simulink model "Simulation_VR"  (R2023a)
settings: Solver=VariableStepAuto  StartTime=0.0  StopTime=15  RelTol=1e-6
values from neighbouring files (symbols this model uses):
  a1 = 1    [main_RR_VR.m]
  a2 = 1    [main_RR_VR.m]
  b = 0.1    [main_RR_VR.m]
  dq0 = [0.0 ; 0.0]    [main_RR_VR.m]
  dq0_d = [0.0; 0.0]    [main_RR_VR.m]
  Il = (1/3)*m1*a1^2    (= 1.66666666667)    [main_RR_VR.m]
  Im = 740e-6    (= 0.00074)    [main_RR_VR.m]
  k_mot = 0.23    [main_RR_VR.m]
  K_pid = 5    [main_RR_VR.m]
  L = 50e-6    (= 5e-05)    [main_RR_VR.m]
  params = [a1, a2, m1, m2, l1, l2, Izz1, Izz2]    [main_RR_VR.m]
  q0 = [0.25 ; 0.25]    [main_RR_VR.m]
  q0_d = [pi/2; -pi/2]    [main_RR_VR.m]
  R = 0.11    [main_RR_VR.m]
  U = diag([1;1; u_min + rand([6,1])*(u_max - u_min)])    [main_RR_VR.m]
undefined symbols (not defined in the file or in its folder): Ks, Lambda, rel_err
settings Model: Creator=Mathew  LastModifiedBy=rvitt
settings SolverCC: AlgebraicLoopSolver=TrustRegion
settings OptimizationCC: ReuseModelBlockBuffer=off
settings DebuggingCC: UnconnectedInputMsg=warning  UnconnectedOutputMsg=warning  UnconnectedLineMsg=warning  ArithmeticOperatorsInVariantConditions=warning
settings ModelReferenceCC: EnableRefExpFcnMdlSchedulingChecks=on
settings SFSimCC: CustomCodeUndefinedFunction=UseInterfaceOnly

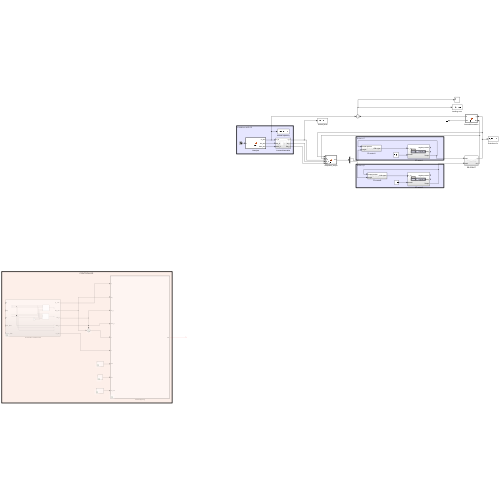
[thumbnail: Simulink's stored preview of the top-level diagram]
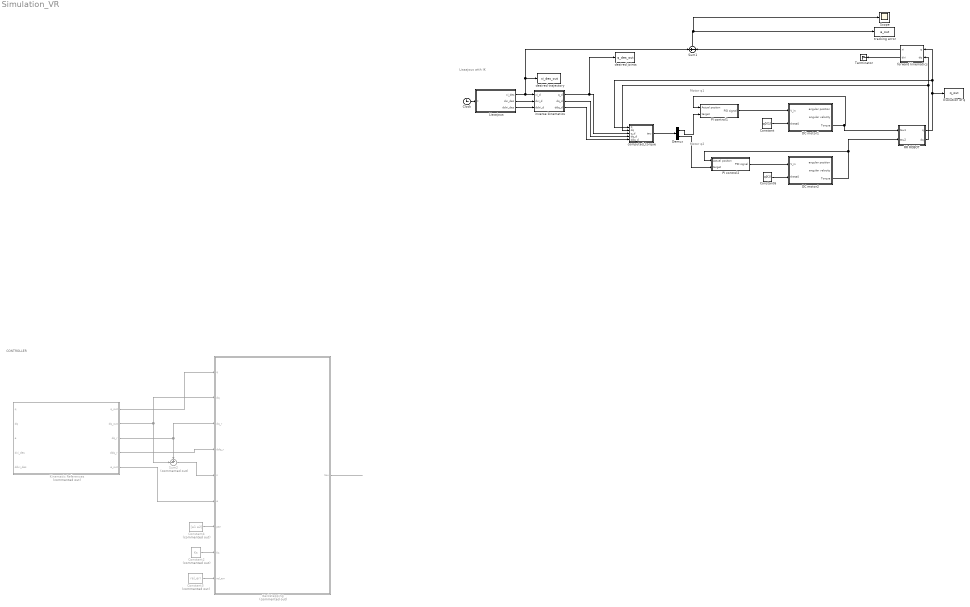
== system Simulation_VR ==
  note: Lissajous with IK
  note: CONTROLLER
  note: Motor q1
  note: Motor q2
  Backstepping : MATLAB Function  Commented=on  TreatAsAtomicUnit=on
  Clock : Clock
  Constant : Constant  Value=q0(1)
  Constant2 : Constant  Commented=on  Value=Ks
  Constant3 : Constant  Commented=on  Value=rel_err
  Constant4 : Constant  Commented=on  Value=[a1 a2]
  Constant6 : Constant  Value=q0(2)
  DC motor1 : Subsystem
  DC motor2 : Subsystem
  Demux : Demux  Outputs=2
  Evolution of q : ToWorkspace  VariableName=q_out  SaveFormat=Timeseries  SampleTime=-1
  Kinematic References : Subsystem  Commented=on
  Lissajous : MATLAB Function  TreatAsAtomicUnit=on
  PI control1 : Subsystem
  PI control2 : Subsystem
  RR ROBOT : Subsystem
  Scope : Scope
  Sum1 : Sum  Inputs=+-
  Sum2 : Sum  Commented=on  Inputs=+-|
  Terminator : Terminator
  computed_torque : MATLAB Function  TreatAsAtomicUnit=on
  desired joints : ToWorkspace  VariableName=q_des_out  SaveFormat=Timeseries  SampleTime=-1
  desired trajectory : ToWorkspace  VariableName=xi_des_out  SaveFormat=Timeseries  SampleTime=-1
  forward kinematics : MATLAB Function  TreatAsAtomicUnit=on
  inverse kinematics : Subsystem
  tracking error : ToWorkspace  VariableName=e_out  SaveFormat=Timeseries  SampleTime=-1
  wires:
  RR ROBOT/1(q) -> computed_torque/1(q), forward kinematics/1(q), Evolution of q/1
  Kinematic References/5(e_out) -> Backstepping/6(e)
  Kinematic References/3(dq_r) -> Backstepping/3(dq_r), Sum2/1
  Constant3/1 -> Backstepping/9(rel_err)
  Kinematic References/2(dq_out) -> Sum2/2, Backstepping/2(dq)
  Kinematic References/1("q_out ") -> Backstepping/1(q)
  Kinematic References/4(ddq_r) -> Backstepping/4(ddq_r)
  Sum2/1 -> Backstepping/5(s)
  Backstepping/1(tau) -> ?
  Constant2/1 -> Backstepping/8(Ks)
  Constant4/1 -> Backstepping/7(par)
  RR ROBOT/2(dq) -> computed_torque/2(dq), forward kinematics/2(dq)
  inverse kinematics/1(q_d) -> computed_torque/3(q_d), desired joints/1
  Clock/1 -> Lissajous/1(t)
  Lissajous/2(dxi_des) -> inverse kinematics/2(dxi_d)
  Lissajous/3(ddxi_des) -> inverse kinematics/3(ddxi_d)
  Lissajous/1(xi_des) -> Sum1/1, desired trajectory/1, inverse kinematics/1(xi_d)
  Sum1/1 -> Scope/1, tracking error/1
  forward kinematics/2(dxi) -> Terminator/1
  forward kinematics/1(xi) -> Sum1/2
  computed_torque/1(tau) -> Demux/1
  inverse kinematics/2(dq_d) -> computed_torque/4(dq_d)
  inverse kinematics/3(ddq_d) -> computed_torque/5(ddq_d)
  PI control1/1(PID signal) -> DC motor1/1(V_in)
  PI control2/1(PID signal) -> DC motor2/1(V_in)
  DC motor1/3(Torque) -> RR ROBOT/1(tau1), PI control1/1(Actual positon)
  Constant/1 -> DC motor1/2(theta0)
  Constant6/1 -> DC motor2/2(theta0)
  DC motor2/3(Torque) -> RR ROBOT/2(tau2), PI control2/1(Actual positon)
  Demux/2 -> PI control2/2(target)
  Demux/1 -> PI control1/2(target)

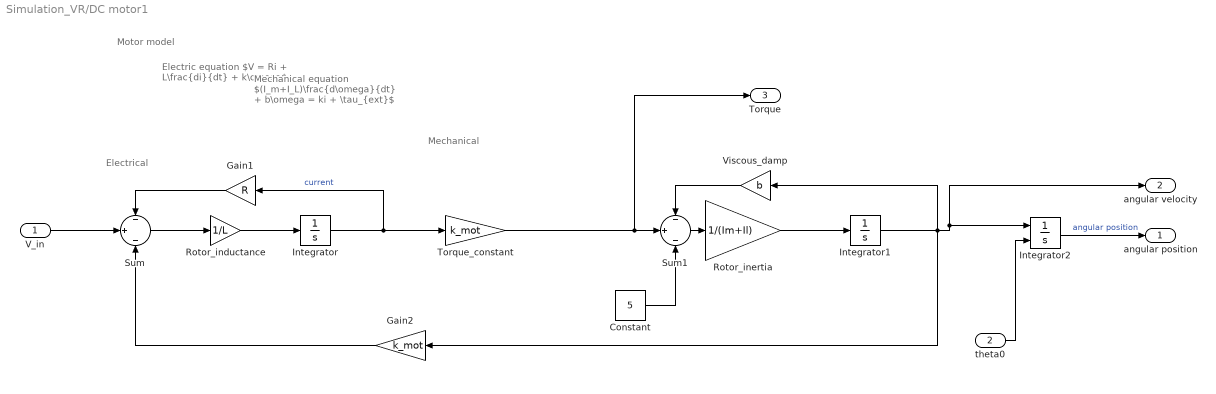
== system Simulation_VR/DC motor1 ==
  note: Electric equation
      | $V = Ri + L\frac{di}{dt} + k\omega$
  note: Mechanical equation
      | $(I_m+I_L)\frac{d\omega}{dt} + b\omega = ki + \tau_{ext}$
  note: Motor model
  note: Electrical
  note: Mechanical
  V_in : Inport
  theta0 : Inport  Port=2
  Constant : Constant  Value=5
  Gain1 : Gain  Gain=R
  Gain2 : Gain  Gain=k_mot
  Integrator : Integrator
  Integrator1 : Integrator
  Integrator2 : Integrator  InitialConditionSource=external
  Rotor_inductance : Gain  Gain=1/L
  Rotor_inertia : Gain  Gain=1/(Im+Il)
  Sum : Sum  Inputs=-|+|-
  Sum1 : Sum  Inputs=-|+|-
  Torque_constant : Gain  Gain=k_mot
  Viscous_damp : Gain  Gain=b
  angular position : Outport
  angular velocity : Outport  Port=2
  Torque : Outport  Port=3
  wires:
  theta0/1 -> Integrator2/2
  Integrator1/1 -> Gain2/1, Integrator2/1, angular velocity/1, Viscous_damp/1
  Torque_constant/1 -> Sum1/2, Torque/1
  Integrator2/1 -> angular position/1  "angular position"
  Gain2/1 -> Sum/3
  Gain1/1 -> Sum/1
  Rotor_inertia/1 -> Integrator1/1
  V_in/1 -> Sum/2
  Rotor_inductance/1 -> Integrator/1
  Sum1/1 -> Rotor_inertia/1
  Viscous_damp/1 -> Sum1/1
  Integrator/1 -> Torque_constant/1, Gain1/1  "current"
  Sum/1 -> Rotor_inductance/1
  Constant/1 -> Sum1/3

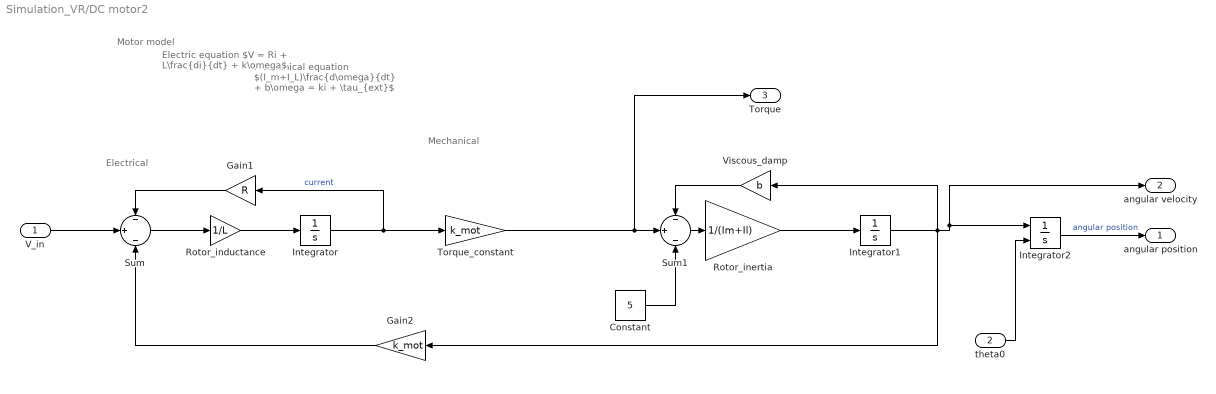
== system Simulation_VR/DC motor2 ==
  note: Mechanical
  note: Electrical
  note: Motor model
  note: Mechanical equation
      | $(I_m+I_L)\frac{d\omega}{dt} + b\omega = ki + \tau_{ext}$
  note: Electric equation
      | $V = Ri + L\frac{di}{dt} + k\omega$
  V_in : Inport
  theta0 : Inport  Port=2
  Constant : Constant  Value=5
  Gain1 : Gain  Gain=R
  Gain2 : Gain  Gain=k_mot
  Integrator : Integrator
  Integrator1 : Integrator
  Integrator2 : Integrator  InitialConditionSource=external
  Rotor_inductance : Gain  Gain=1/L
  Rotor_inertia : Gain  Gain=1/(Im+Il)
  Sum : Sum  Inputs=-|+|-
  Sum1 : Sum  Inputs=-|+|-
  Torque_constant : Gain  Gain=k_mot
  Viscous_damp : Gain  Gain=b
  angular position : Outport
  angular velocity : Outport  Port=2
  Torque : Outport  Port=3
  wires:
  Sum/1 -> Rotor_inductance/1
  Integrator/1 -> Gain1/1, Torque_constant/1  "current"
  Viscous_damp/1 -> Sum1/1
  Sum1/1 -> Rotor_inertia/1
  Rotor_inductance/1 -> Integrator/1
  V_in/1 -> Sum/2
  Rotor_inertia/1 -> Integrator1/1
  Gain1/1 -> Sum/1
  Gain2/1 -> Sum/3
  Integrator2/1 -> angular position/1  "angular position"
  Torque_constant/1 -> Torque/1, Sum1/2
  Integrator1/1 -> Viscous_damp/1, angular velocity/1, Integrator2/1, Gain2/1
  theta0/1 -> Integrator2/2
  Constant/1 -> Sum1/3

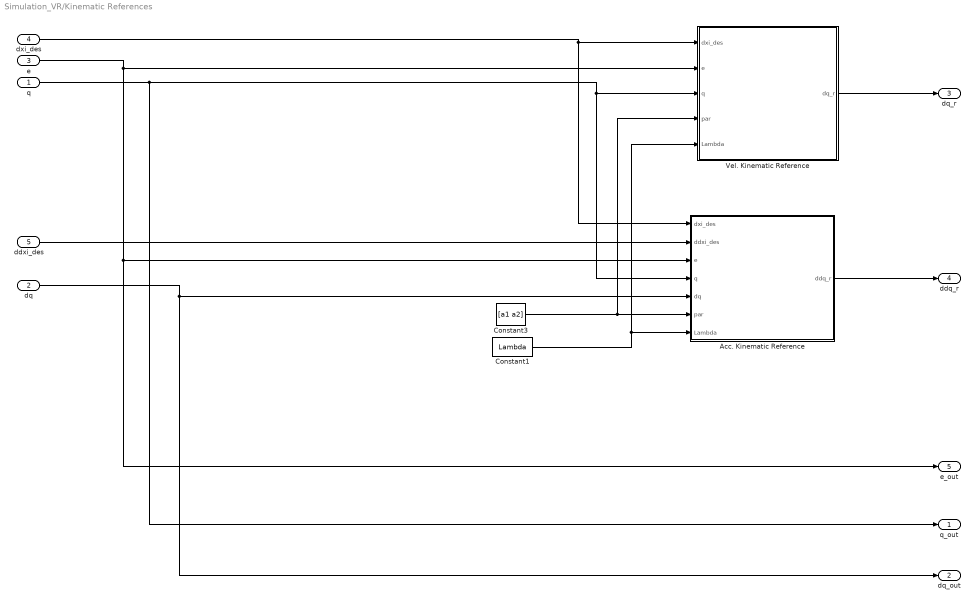
== system Simulation_VR/Kinematic References ==
  q : Inport
  dq : Inport  Port=2
  e : Inport  Port=3
  dxi_des : Inport  Port=4
  ddxi_des : Inport  Port=5
  Acc. Kinematic Reference : MATLAB Function  TreatAsAtomicUnit=on
  Constant1 : Constant  Value=Lambda
  Constant3 : Constant  Value=[a1 a2]
  "Vel. Kinematic Reference " : MATLAB Function  TreatAsAtomicUnit=on
  "q_out " : Outport  VectorParamsAs1DForOutWhenUnconnected=off
  dq_out : Outport  Port=2  VectorParamsAs1DForOutWhenUnconnected=off
  dq_r : Outport  Port=3  VectorParamsAs1DForOutWhenUnconnected=off
  ddq_r : Outport  Port=4  VectorParamsAs1DForOutWhenUnconnected=off
  e_out : Outport  Port=5  VectorParamsAs1DForOutWhenUnconnected=off
  wires:
  ddxi_des/1 -> Acc. Kinematic Reference/2(ddxi_des)
  e/1 -> e_out/1, Acc. Kinematic Reference/3(e), "Vel. Kinematic Reference "/2(e)
  dxi_des/1 -> Acc. Kinematic Reference/1(dxi_des), "Vel. Kinematic Reference "/1(dxi_des)
  Constant1/1 -> "Vel. Kinematic Reference "/5(Lambda), Acc. Kinematic Reference/7(Lambda)
  "Vel. Kinematic Reference "/1(dq_r) -> dq_r/1
  dq/1 -> dq_out/1, Acc. Kinematic Reference/5(dq)
  q/1 -> "q_out "/1, Acc. Kinematic Reference/4(q), "Vel. Kinematic Reference "/3(q)
  Constant3/1 -> "Vel. Kinematic Reference "/4(par), Acc. Kinematic Reference/6(par)
  Acc. Kinematic Reference/1(ddq_r) -> ddq_r/1

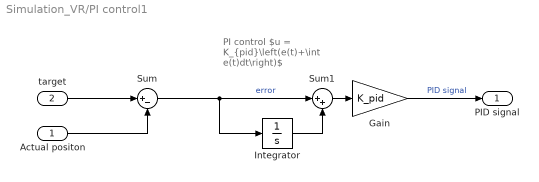
== system Simulation_VR/PI control1 ==
  note: PI control
      | $u = K_{pid}\left(e(t)+\int e(t)dt\right)$
  Actual positon : Inport
  target : Inport  Port=2
  Gain : Gain  Gain=K_pid
  Integrator : Integrator
  Sum : Sum  Inputs=|+-
  Sum1 : Sum  Inputs=|++
  PID signal : Outport
  wires:
  Actual positon/1 -> Sum/2
  Sum1/1 -> Gain/1
  Gain/1 -> PID signal/1  "PID signal"
  Sum/1 -> Integrator/1, Sum1/1  "error"
  target/1 -> Sum/1
  Integrator/1 -> Sum1/2

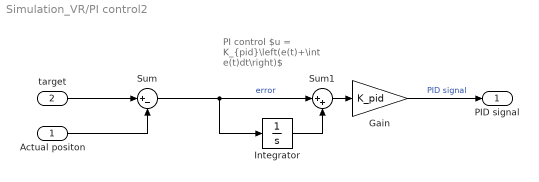
== system Simulation_VR/PI control2 ==
  note: PI control
      | $u = K_{pid}\left(e(t)+\int e(t)dt\right)$
  Actual positon : Inport
  target : Inport  Port=2
  Gain : Gain  Gain=K_pid
  Integrator : Integrator
  Sum : Sum  Inputs=|+-
  Sum1 : Sum  Inputs=|++
  PID signal : Outport
  wires:
  Integrator/1 -> Sum1/2
  target/1 -> Sum/1
  Sum/1 -> Sum1/1, Integrator/1  "error"
  Gain/1 -> PID signal/1  "PID signal"
  Sum1/1 -> Gain/1
  Actual positon/1 -> Sum/2

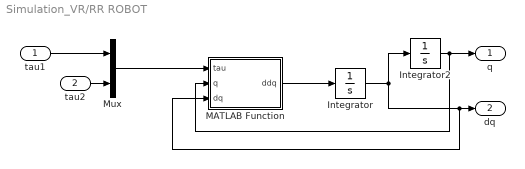
== system Simulation_VR/RR ROBOT ==
  tau1 : Inport
  tau2 : Inport  Port=2
  Integrator : Integrator  InitialCondition=dq0
  Integrator2 : Integrator  InitialCondition=q0
  MATLAB Function : MATLAB Function  TreatAsAtomicUnit=on
  Mux : Mux  Inputs=2
  q : Outport  PortDimensions=[2,1]
  dq : Outport  Port=2  PortDimensions=[2,1]
  wires:
  Mux/1 -> MATLAB Function/1(tau)
  MATLAB Function/1(ddq) -> Integrator/1
  Integrator/1 -> Integrator2/1, MATLAB Function/3(dq), dq/1
  Integrator2/1 -> MATLAB Function/2(q), q/1
  tau1/1 -> Mux/1
  tau2/1 -> Mux/2

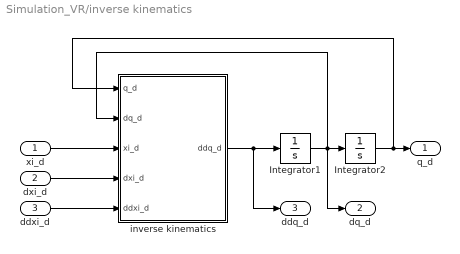
== system Simulation_VR/inverse kinematics ==
  xi_d : Inport
  dxi_d : Inport  Port=2
  ddxi_d : Inport  Port=3
  Integrator1 : Integrator  InitialCondition=dq0_d
  Integrator2 : Integrator  InitialCondition=q0_d
  inverse kinematics : MATLAB Function  TreatAsAtomicUnit=on
  q_d : Outport  PortDimensions=[2,1]
  dq_d : Outport  Port=2  PortDimensions=[2,1]
  ddq_d : Outport  Port=3  PortDimensions=[2,1]
  wires:
  inverse kinematics/1(ddq_d) -> Integrator1/1, ddq_d/1
  Integrator2/1 -> inverse kinematics/1(q_d), q_d/1
  ddxi_d/1 -> inverse kinematics/5(ddxi_d)
  dxi_d/1 -> inverse kinematics/4(dxi_d)
  xi_d/1 -> inverse kinematics/3(xi_d)
  Integrator1/1 -> inverse kinematics/2(dq_d), dq_d/1, Integrator2/1

== matlab function Simulation_VR/forward kinematics ==
  data: q input; xi output; dq input; params parameter; dxi output
function [xi, dxi] = fcn(q, dq, params)

[xi, dxi] = RR_forward_kinematics(q, dq, params);

end

== matlab function Simulation_VR/computed_torque ==
  data: q input; tau output; dq input; q_d input; dq_d input; ddq_d input; params parameter; U parameter
function tau  = fcn(q, dq, q_d, dq_d, ddq_d, params, U)

% uncertanties
% params = params;

% robot matrix
M = get_M(q,params);
C = get_C(q,dq,params);
G = get_G(q, params);

% errors computation
e = q_d - q;
de = dq_d - dq;

% gains
kp = 5;
kv = 3;

% computed torque
tau = M*(ddq_d + kv*de + kp*e) + C*dq + G;

% robustness
A = [zeros(2,2) eye(2,2);...
    -kp*eye(2,2) -kv*eye(2,2)];

B = [zeros(2,2); eye(2,2)];

coder.extrinsic('lyap');
P = zeros(4,4);
P = lyap(A', eye(4,4));

x = [e; de];

w = B'*P*x;
rho = 10;
eps = 0.001;

delta = rho*w / (sqrt(w'*w + eps));

tau = tau + M*delta;

== matlab function Simulation_VR/RR ROBOT/MATLAB Function ==
  data: tau input; ddq output; q input; dq input; params parameter
function ddq  = fcn(tau, q, dq, params)

% get the matrix for the model
M = get_M(q,params);
C = get_C(q,dq,params);
G = get_G(q, params);

% inversion of dinamic equations (M def+)
ddq = inv(M)*(tau-C*dq-G);

== matlab function Simulation_VR/Backstepping ==
  data: q input; dq input; dq_r input; tau output; ddq_r input; s input; e input; par input; Ks input; rel_err input
function tau = backstepping(q, dq, dq_r, ddq_r, s, e, par, Ks, rel_err)

coder.extrinsic('disp');

% Get dynamic matrices
M = RR_mass_matrix(q);
C = RR_coriolis_matrix(q, dq);
G = RR_gravity_vector(q);

% % Adding uncertainty
% M = M.*(1 + rel_err);
% C = C.*(1 + rel_err);
% G = G.*(1 + rel_err);

% Get Jacobian
J = RR_jacobian(q, par);

% Control law
tau = M*ddq_r + C*dq_r + G + Ks*s + J.'*e;

== matlab function Simulation_VR/Kinematic References/Acc. Kinematic Reference ==
  data: dxi_des input; ddq_r output; ddxi_des input; e input; q input; dq input; par input; Lambda input
function ddq_r = acc_kinematic_reference(dxi_des, ddxi_des, e, q, dq, par, Lambda)

coder.extrinsic('disp');

J = zeros(2,2);
dJ = zeros(2,2);

% Computing jacobian and derivative
J = RR_jacobian(q, par);
dJ = RR_diff_jacobian(q, dq, par);

ddq_r = inv(J) * (ddxi_des + Lambda*dxi_des - Lambda*J*dq) ...
- inv(J)*dJ*inv(J)*(dxi_des + Lambda*e);
end

== matlab function Simulation_VR/Kinematic References/Vel. Kinematic Reference  ==
  data: dxi_des input; dq_r output; e input; q input; par input; Lambda input
function dq_r = vel_kinematic_reference(dxi_des, e, q, par, Lambda)

% Computing jacobian
J = RR_jacobian(q, par);

dq_r = inv(J) * (dxi_des + Lambda*e);
end

== matlab function Simulation_VR/Lissajous ==
  data: t input; xi_des output size=[2,1]; dxi_des output size=[2,1]; ddxi_des output size=[2,1]; par_traj parameter
function [xi_des, dxi_des, ddxi_des] = lissajous(t, par_traj)

A = par_traj.A;
B = par_traj.B;
a = par_traj.a;
b = par_traj.b;
d = par_traj.d;
xi0 = par_traj.xi0;

xi_des = [A*sin(a*t+d); B*sin(b*t)] + xi0;
dxi_des = [A*a*cos(a*t+d); B*b*cos(b*t)];
ddxi_des = [-A*a^2*sin(a*t+d); -B*b^2*sin(b*t)];

== matlab function Simulation_VR/inverse kinematics/inverse kinematics ==
  data: q_d input; dq_d input; xi_d input; dxi_d input; ddxi_d input; ddq_d output; params parameter
function ddq_d = fcn(q_d, dq_d, xi_d, dxi_d, ddxi_d, params)

% jacobian
J = get_J(q_d, params);
% jacobian derivative
J_dot = get_J_dot(q_d, dq_d, params);
% pseudoinverse
pinv_J = pinv(J);
% forward kinematics
[xi_curr, dxi_curr] = RR_forward_kinematics(q_d, dq_d, params);

% second order CLIK
Kp = 100;
Kv = 30;
ddq_d = pinv_J * (ddxi_d - J_dot * dq_d + Kv*(dxi_d-dxi_curr) + Kp*(xi_d-xi_curr));
